simulink model "ModeloManual2"  (R2022a)
settings: Solver=VariableStepAuto  StartTime=0.0  StopTime=10.0  RelTol=1e-3
values from neighbouring files (symbols this model uses):
  a = 0.2    [Data.m]
  b = 0.15    [Data.m]
  m3 = pinv(m2)    [Data.m]
  N = 4365    [GraficasVelocidades.m]    (also in Prueba_Liapunov.m = length(p_X); WaypointsToTrayectory.m = length(X))
  R = 0.16/2    (= 0.08)    [Data.m]
  X = M(:,1)    [WaypointsToTrayectory.m]
  Y = M(:, 2)    [WaypointsToTrayectory.m]
undefined symbols (not defined in the file or in its folder): c, Z
libraries: sm_lib x34, nesl_utility x15, fl_lib x9, ee_lib x1, robotalgslib x1, mobileRoboticsLib x1
(part 2 of 2)

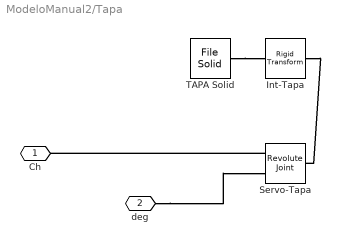
== system ModeloManual2/Tapa ==
  Int-Tapa : sm_lib/Frames and Transforms/Rigid Transform  TranslationMethod=Cartesian  TranslationStandardOffset=0  TranslationLengthUnit=mm  TranslationStandardAxis=+Z  TranslationCartesianOffset=[177 140 12.5]  TranslationROffset=0  TranslationROffsetUnits=m  TranslationZOffset=0  TranslationZOffsetUnits=m  TranslationThetaOffset=0  TranslationThetaOffsetUnits=deg  RotationMethod=StandardAxis  RotationAngleUnits=deg  RotationStandardAxis=+X  RotationAngle=90  RotationArbitraryAxis=[0 0 1]  FollAlignAxisA=+X  BaseAlignAxisA=+Y  FollAlignAxisB=+Y  BaseAlignAxisB=+Z  RotationSequenceAxes=FollowerAxes  RotationSequence=XYX  RotationSequenceAngles=[0 0 0]  RotationSequenceAnglesUnits=deg  RotationMatrix=[1 0 0; 0 1 0; 0 0 1]
  Servo-Tapa : sm_lib/Joints/Revolute Joint  JointMode=Normal  SenseConstraintForce=off  SenseConstraintForceX=off  SenseConstraintForceY=off  SenseConstraintForceZ=off  SenseConstraintTorque=off  SenseConstraintTorqueX=off  SenseConstraintTorqueY=off  SenseConstraintTorqueZ=off  SenseTotalForce=off  SenseTotalForceX=off  SenseTotalForceY=off  SenseTotalForceZ=off  SenseTotalTorque=off  SenseTotalTorqueX=off  SenseTotalTorqueY=off  SenseTotalTorqueZ=off  CompositeWrenchDir=FollowerOnBase  CompositeWrenchFrame=BaseFrame  EquilibriumPosition=0  EquilibriumPositionUnits=deg  SpringStiffness=0  SpringStiffnessUnits=N*m/deg  DampingCoefficient=0  DampingCoefficientUnits=N*m/(deg/s)  TorqueActuationMode=ComputedTorque  MotionActuationMode=InputMotion  SensePosition=off  SenseVelocity=off  SenseAcceleration=off  SenseTorqueForce=off  SenseLowerLimitTorqueForce=off  SenseUpperLimitTorqueForce=off  LowerLimitSpecify=on  LowerLimitBound=-pi/2  LowerLimitBoundUnits=deg  LowerLimitStiffness=1e4  LowerLimitStiffnessUnits=N*m/deg  LowerLimitDamping=10  LowerLimitDampingUnits=N*m/(deg/s)  LowerLimitTransitionRegionWidth=0.1  LowerLimitTransitionRegionWidthUnits=deg  UpperLimitSpecify=on  UpperLimitBound=0  UpperLimitBoundUnits=deg  UpperLimitStiffness=1e4  UpperLimitStiffnessUnits=N*m/deg  UpperLimitDamping=10  UpperLimitDampingUnits=N*m/(deg/s)  UpperLimitTransitionRegionWidth=0.1  UpperLimitTransitionRegionWidthUnits=deg  PositionTargetSpecify=off  PositionTargetPriority=High  PositionTargetValue=0  PositionTargetValueUnits=deg  VelocityTargetSpecify=off  VelocityTargetPriority=High  VelocityTargetValue=0  VelocityTargetValueUnits=deg/s
  TAPA Solid : sm_lib/Body Elements/File Solid  ExtGeomFileName=TapaOriented_ipt_dee1459.STEP  UnitType=FromFile  ExtGeomFileUnits=m  StepReaderType=HEX  ExportConvexHullGeometry=off  InertiaType=CalculateFromGeometry  Mass=2  MassUnits=kg  CenterOfMass=[0 0 0]  CenterOfMassUnits=m  MomentsOfInertia=[1 1 1]  MomentsOfInertiaUnits=kg*m^2  ProductsOfInertia=[0 0 0]  ProductsOfInertiaUnits=kg*m^2  BasedOnType=Mass  Density=1000  DensityUnits=kg/m^3  DoExposeReferenceFrame=on  SerializedFrames=<Frames/>  GraphicType=FromGeometry  MarkerShape=Sphere  MarkerSize=10  GraphicVisPropType=SimpleVisualProperties  GraphicDiffuseColor=[0.5 0.5 0.5]  GraphicSpecularColor=[0.5 0.5 0.5 1.0]  GraphicAmbientColor=[0.15 0.15 0.15 1.0]  GraphicEmissiveColor=[0.0 0.0 0.0 1.0]  GraphicShininess=75  GraphicOpacity=1.0
  Ch : PMIOPort  Side=Left
  deg : PMIOPort  Port=2  Side=Right
  connections:
  TAPA Solid/RConn1 -- Int-Tapa/LConn1
  Int-Tapa/RConn1 -- Servo-Tapa/RConn1
  deg/RConn1 -- Servo-Tapa/LConn2
  Servo-Tapa/LConn1 -- Ch/RConn1

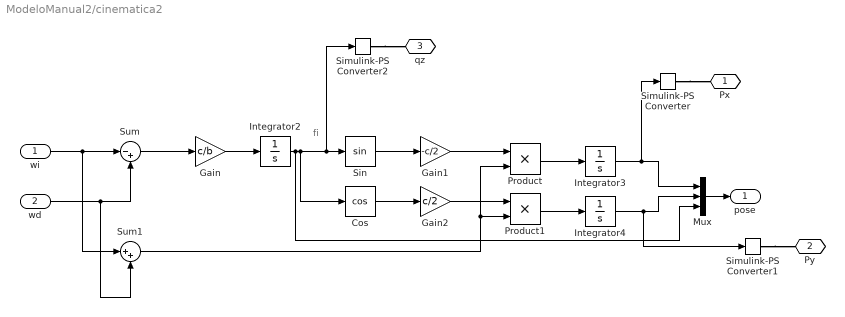
== system ModeloManual2/cinematica2 ==
  note: fi
  wi : Inport
  wd : Inport  Port=2
  Cos : Trigonometry  Operator=cos
  Gain : Gain  Gain=c/b
  Gain1 : Gain  Gain=-c/2
  Gain2 : Gain  Gain=c/2
  Integrator2 : Integrator
  Integrator3 : Integrator
  Integrator4 : Integrator
  Mux : Mux  Inputs=3
  Product : Product
  Product1 : Product
  Simulink-PS Converter : nesl_utility/Simulink-PS Converter  PhysicalDomain=network_engine_domain  SubClassName=ps_input  LeftPortType=input  RightPortType=output  PseudoPeriodic=off  Frequencies=[]  NoiseDistribution=none  NoiseParameters=[]  Unit=m  AffineConversion=off  FilteringAndDerivatives=filter  SimscapeFilterOrder=2  InputFilterTimeConstant=0.001  UdotUserProvided=0
      settings: SourceProductBaseCode=SS,PW,VE
  Simulink-PS Converter1 : nesl_utility/Simulink-PS Converter  PhysicalDomain=network_engine_domain  SubClassName=ps_input  LeftPortType=input  RightPortType=output  PseudoPeriodic=off  Frequencies=[]  NoiseDistribution=none  NoiseParameters=[]  Unit=m  AffineConversion=off  FilteringAndDerivatives=filter  SimscapeFilterOrder=2  InputFilterTimeConstant=0.001  UdotUserProvided=0
      settings: SourceProductBaseCode=SS,PW,VE
  Simulink-PS Converter2 : nesl_utility/Simulink-PS Converter  PhysicalDomain=network_engine_domain  SubClassName=ps_input  LeftPortType=input  RightPortType=output  PseudoPeriodic=off  Frequencies=[]  NoiseDistribution=none  NoiseParameters=[]  Unit=rad  AffineConversion=off  FilteringAndDerivatives=filter  SimscapeFilterOrder=2  InputFilterTimeConstant=0.001  UdotUserProvided=0
      settings: SourceProductBaseCode=SS,PW,VE
  Sin : Trigonometry
  Sum : Sum  Inputs=|-+
  Sum1 : Sum  Inputs=|++
  Px : PMIOPort  Side=Right
  Py : PMIOPort  Port=2  Side=Right
  qz : PMIOPort  Port=3  Side=Right
  pose : Outport
  wires:
  Sum1/1 -> Product1/2, Product/2
  Gain1/1 -> Product/1
  wi/1 -> Sum1/1, Sum/1
  wd/1 -> Sum1/2, Sum/2
  Product/1 -> Integrator3/1
  Cos/1 -> Gain2/1
  Gain/1 -> Integrator2/1
  Sum/1 -> Gain/1
  Product1/1 -> Integrator4/1
  Sin/1 -> Gain1/1
  Gain2/1 -> Product1/1
  Integrator3/1 -> Simulink-PS Converter/1, Mux/1
  Mux/1 -> pose/1
  Integrator4/1 -> Simulink-PS Converter1/1, Mux/2
  Integrator2/1 -> Mux/3, Cos/1, Simulink-PS Converter2/1, Sin/1
  connections:
  Simulink-PS Converter/RConn1 -- Px/RConn1
  Simulink-PS Converter1/RConn1 -- Py/RConn1
  Simulink-PS Converter2/RConn1 -- qz/RConn1

== matlab function ModeloManual2/Direct-Kinematics/MATLAB Function ==
  data: xp output; yp output; wr input; wl input; r input; c input; a input; o output; or input
function [xp,yp,o] = fcn(wr,wl,r,c,a,or)

o= or;

v1= c*cos(o) - 2*a*sin(o);
v2= c*cos(o) + 2*a*sin(o);
v3= c*sin(o) + 2*a*cos(o);
v4= c*sin(o) - 2*a*cos(o);

xp=(r/(2*c))*(v1*wr+v2*wl);
yp=(r/(2*c))*(v3*wr+v4*wl);
